simulink model "WHEELSPEEDTEST"  (R2024b)
settings: Solver=ode4  StartTime=0.0  StopTime=T_SIM  FixedStep=T_s  RelTol=1e-3
values from neighbouring files (symbols this model uses):
  control_par = [1.5, 1.5, 0.3]    [TASK1_Script.m]    (also in TASK2_LAB_SCRIPT.m = update_control_par(controller_index); TASK2_Scirpt.m = [k1, k2,b]; TASK3_Script.m = [k1, k2,b])
  d = d_actual    (= 0.1604)    [TASK1_Script.m]    (also in TASK2_LAB_SCRIPT.m; TASK2_Scirpt.m; TASK3_Script.m)
  D = diag([0.8e-3, 0.8e-3, 5e-3, 0.0175/6, 0.0175/6, 0.0175/6*T_s, 0.0175/6*T_s].^2)    [TASK1_Script.m]    (also in TASK2_LAB_SCRIPT.m; TASK2_Scirpt.m; TASK3_Script.m)
  d_actual = 0.16040    (= 0.1604)    [TASK1_Script.m]    (also in TASK2_LAB_SCRIPT.m; TASK2_Scirpt.m; TASK3_Script.m)
  H_enc = [0, 0, 0, 1, 0, 0, 0 ... (first row only)    [TASK1_Script.m]    (also in TASK2_LAB_SCRIPT.m; TASK2_Scirpt.m; TASK3_Script.m)
  H_gyro = [0, 0, 0, 0, 0, -r_actual/d_actual, r_actual/d_actual]    [TASK1_Script.m]    (also in TASK2_LAB_SCRIPT.m; TASK2_Scirpt.m; TASK3_Script.m)
  H_motion_cap = [1, 0, 0, 0, 0, 0, 0 ... (first row only)    [TASK1_Script.m]    (also in TASK2_LAB_SCRIPT.m; TASK2_Scirpt.m; TASK3_Script.m)
  omega_M = 10    [TASK1_Script.m]    (also in TASK2_LAB_SCRIPT.m; TASK2_Scirpt.m; TASK3_Script.m)
  P_INIT_EKF = diag([0.1, 0.1, 0.2, 0.0175/6, 0.0175/6, 0.0175/6*T_s, 0.0175/6*T_s].^2)    [TASK1_Script.m]    (also in TASK2_LAB_SCRIPT.m; TASK2_Scirpt.m; TASK3_Script.m)
  p_loss = 0.9    [TASK3_Script.m]
  PHI_INIT = [0;0]    [TASK1_Script.m]    (also in TASK2_LAB_SCRIPT.m; TASK2_Scirpt.m; TASK3_Script.m)
  q_d = [-1.6; -1.1; 0]    [TASK1_Script.m]
  Q_INIT = Q_INIT_1    [TASK1_Script.m]    (also in TASK2_LAB_SCRIPT.m = [-1.6;-1.1;0]; TASK2_Scirpt.m = [-1.6;-1.1;0]; TASK3_Script.m = [x7; y4; 0])
  r = r_actual    (= 0.03293)    [TASK1_Script.m]    (also in TASK2_LAB_SCRIPT.m; TASK2_Scirpt.m; TASK3_Script.m)
  R_3 = diag(([sigma_motion_capture, sigma_motion_capture, sigma_motion_capture,               sigma_enc, sigma_enc, sigma_imu]).^2)    [TASK1_Script.m]    (also in TASK2_LAB_SCRIPT.m; TASK2_Scirpt.m; TASK3_Script.m)
  r_actual = 0.03293    [TASK1_Script.m]    (also in TASK2_LAB_SCRIPT.m; TASK2_Scirpt.m; TASK3_Script.m)
  T_s = 0.04    [TASK1_Script.m]    (also in TASK2_LAB_SCRIPT.m; TASK2_Scirpt.m; TASK3_Script.m; plot_4_wheel_velocities.m)
  tol = 0.025    [TASK1_Script.m]
  Z_INIT_EKF = [Q_INIT; 0; 0; 0; 0]    [TASK1_Script.m]    (also in TASK2_LAB_SCRIPT.m; TASK2_Scirpt.m; TASK3_Script.m)
undefined symbols (not defined in the file or in its folder): X, Y
libraries: robotlib x6, sharedtransform x2, dspsigops x1
settings Model: Creator=tomailoren  LastModifiedBy=llp
settings OptimizationCC: DefaultParameterBehavior=Inlined  EnhancedBackFolding=on  PassReuseOutputArgsAs=Individual arguments  ZeroExternalMemoryAtStartup=off  ZeroInternalMemoryAtStartup=off  MaxStackSize=64  OptimizeBlockOrder=speed  DifferentSizesBufferReuse=on  OptimizationCustomize=off  EfficientTunableParamExpr=on
settings DebuggingCC: ParameterTunabilityLossMsg=error
settings HardwareCC: ProdBitPerPointer=32  ProdBitPerSizeT=32  ProdBitPerPtrDiffT=32  ProdLargestAtomicFloat=None  ProdIntDivRoundTo=Undefined  ProdEndianess=Unspecified  ProdWordSize=32  ProdHWDeviceType=Generic->Unspecified (assume 32-bit Generic)
settings SFSimCC: MATLABDynamicMemAlloc=off
settings RTWCC: Description=Embedded Coder  SystemTargetFile=ert.tlc  HardwareBoard=Robot Operating System (ROS)  TLCOptions="-aInlineSetEventsForThisBaseRateFcn=TLC_FALSE -aSuppressMultiTaskScheduler=TLC_FALSE  -aRateBasedStepFcn=0"  TemplateMakefile=ert_default_tmf  Toolchain=Catkin  TargetLang=C++
settings CodeAppCC: ForceParamTrailComments=on  IgnoreCustomStorageClasses=off  OperatorAnnotations=on  SimulinkDataObjDesc=on  SFDataObjDesc=on  InsertBlockDesc=on

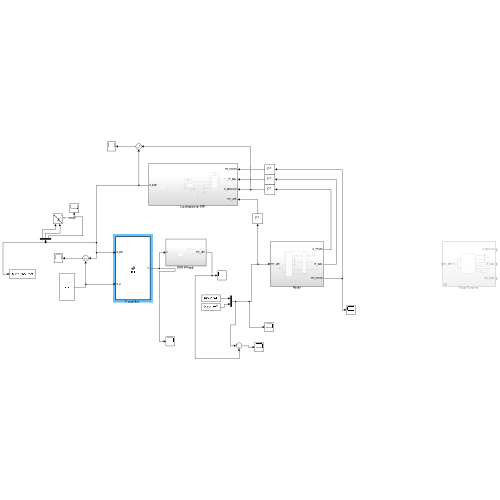
[thumbnail: Simulink's stored preview of the top-level diagram]
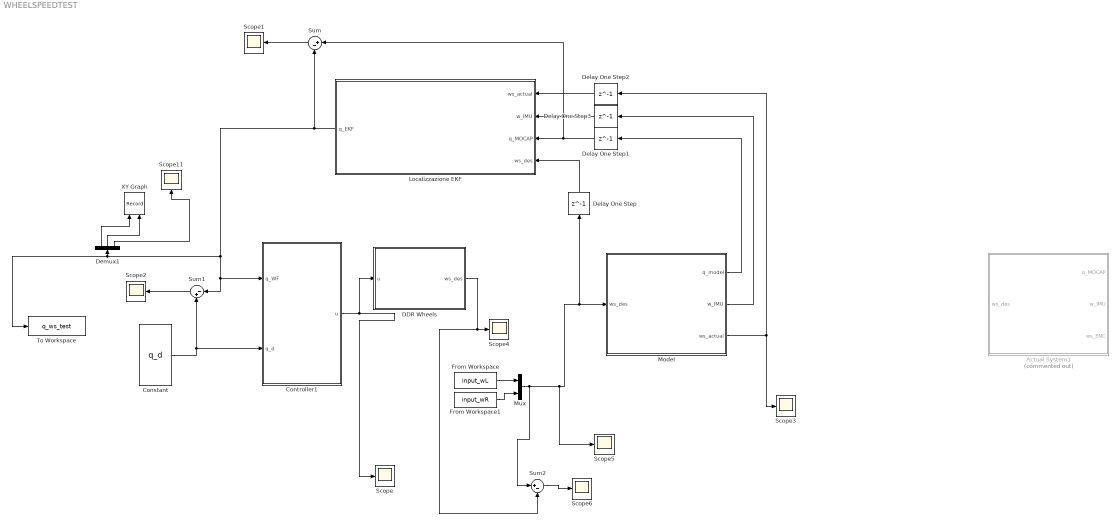
== system WHEELSPEEDTEST ==
  Actual System1 : Subsystem  Commented=on
  Constant : Constant  Value=q_d
  Controller1 : MATLAB Function  TreatAsAtomicUnit=on
  DDR Wheels : Subsystem
  Delay One Step : Delay  DelayLength=1  InitialCondition=[0;0]  SampleTime=T_s
  Delay One Step1 : Delay  DelayLength=1  InitialCondition=Q_INIT  SampleTime=T_s
  Delay One Step2 : Delay  DelayLength=1  InitialCondition=[0;0]  SampleTime=T_s
  Delay One Step3 : Delay  DelayLength=1  InitialCondition=0  SampleTime=T_s
  Demux1 : Demux  Outputs=3
  From Workspace : FromWorkspace  VariableName=input_wL
  From Workspace1 : FromWorkspace  VariableName=input_wR
  Localizzazione EKF : Subsystem
  Model : Subsystem
  Mux : Mux  Inputs=2
  Scope{,1..6,11} (8 alike) : Scope
  Sum : Sum  Inputs=|+-
  Sum1 : Sum  Inputs=|-+
  Sum2 : Sum  Inputs=|+-
  To Workspace : ToWorkspace  VariableName=q_ws_test  SaveFormat=Structure With Time  SampleTime=-1
  XY Graph : Record  FileSettingsInternal="{\"entries\":[{\"content\":{\"excelSettings\":{\"content\":{},\"type\":\"Streamout.ExcelSettings\"}},\"type\":\"Streamout.FileSettingStorage\",\"uuid\":\"\"}],\"packageUris\":[\"http:\\/\\/schema.mathworks.com\\/mf0\\/streamout_blocks\\/R2020a\"],\"version\":\"1.0\"}"  Layout=[1 1]  SignalsInternal="{\"entries\":[{\"content\":{\"signals\":[{\"content\":{\"blockPath\":[],\"dimensions\":[1,1],\"domain\":\"\",\"lineColor\":\"#a2142f\",\"plots\":[ 1 ],\"port\":1,\"signalID\":1,\"signalName\":\"Demux1:1\"},\"type\":\"RecordBlkView.Signal\",\"uuid\":\"\"},{\"content\":{\"blockPath\":[],\"dimensions\":[1,1],\"domain\":\"\",\"lineColor\":\"#139fff\",\"plots\":[ 1 ],\"port\":2,\"signalID\":2,\"signalName\":\"Demux1:2\"},\"type\":\"RecordBlkView.Signal\",\"uuid\":\"\"}]},\"type\":\"RecordBlkView.InputSignals\",\"uuid\":\"\"}],\"packageUris\":[\"http:\\/\\/schema.mathworks.com\\/mf0\\/streamout_blocks\\/R2020a\"],\"version\":\"1.0\"}"  VisualizationBindings="{\"xyplotplugin\":{\"info\":[{\"series\":[{\"bindingParametersList\":[{\"parameter\":\"X-Axis\",\"signalID\":1,\"signalName\":\"Demux1:1\"},{\"parameter\":\"Y-Axis\",\"signalID\":2,\"signalName\":\"Demux1:2\"}],\"seriesID\":0}],\"subplotID\":1}]}}"  CompatibilityTag=XY
  wires:
  Controller1/1(u) -> Scope/1, DDR Wheels/1(u)
  Localizzazione EKF/1(q_EKF) -> Sum/2, Sum1/1, Controller1/1(q_WF), To Workspace/1, Demux1/1
  Model/1(q_model) -> Delay One Step1/1
  Model/3(ws_actual) -> Scope3/1, Delay One Step2/1
  Model/2(w_IMU) -> Delay One Step3/1
  Delay One Step/1 -> Localizzazione EKF/4(ws_des)
  Constant/1 -> Sum1/2, Controller1/2(q_d)
  Demux1/1 -> XY Graph/1
  Demux1/2 -> XY Graph/2
  Demux1/3 -> Scope11/1
  Delay One Step1/1 -> Sum/1, Localizzazione EKF/3(q_MOCAP)
  Delay One Step2/1 -> Localizzazione EKF/1(ws_actual)
  Delay One Step3/1 -> Localizzazione EKF/2(w_IMU)
  Sum/1 -> Scope1/1
  Sum1/1 -> Scope2/1
  DDR Wheels/1(ws_des) -> Sum2/2, Scope4/1
  Mux/1 -> Sum2/1, Scope5/1, Delay One Step/1, Model/1(ws_des)
  From Workspace/1 -> Mux/1
  From Workspace1/1 -> Mux/2
  Sum2/1 -> Scope6/1

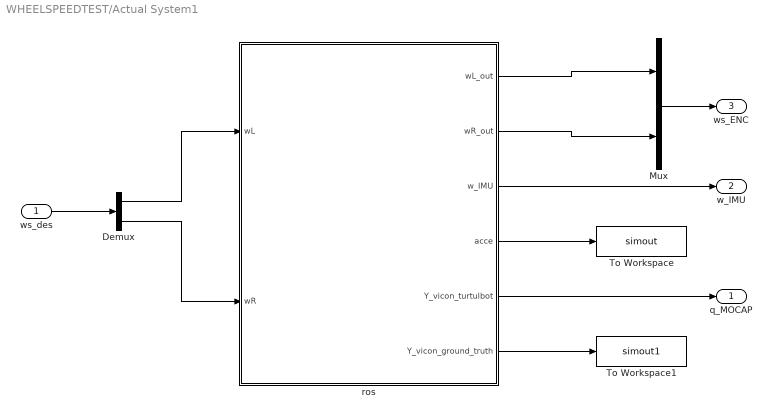
== system WHEELSPEEDTEST/Actual System1 ==
  ws_des : Inport
  Demux : Demux  Outputs=2
  Mux : Mux  Inputs=2
  To Workspace : ToWorkspace  VariableName=simout  SaveFormat=Timeseries  SampleTime=-1
  To Workspace1 : ToWorkspace  VariableName=simout1  SaveFormat=Timeseries  SampleTime=-1
  ros : Subsystem
  q_MOCAP : Outport
  w_IMU : Outport  Port=2
  ws_ENC : Outport  Port=3
  wires:
  ros/2(wR_out) -> Mux/2
  ros/4(acce) -> To Workspace/1
  ros/5(Y_vicon_turtulbot) -> q_MOCAP/1
  ros/1(wL_out) -> Mux/1
  ros/3(w_IMU) -> w_IMU/1
  ws_des/1 -> Demux/1
  Demux/1 -> ros/1(wL)
  Demux/2 -> ros/2(wR)
  Mux/1 -> ws_ENC/1
  ros/6(Y_vicon_ground_truth) -> To Workspace1/1

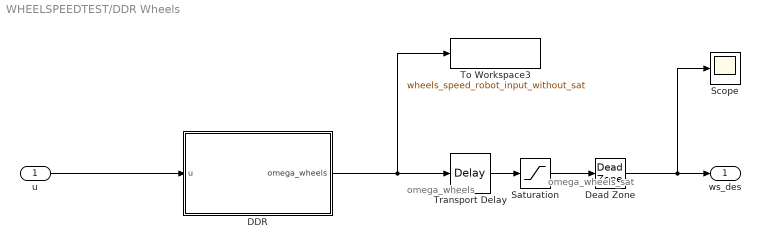
== system WHEELSPEEDTEST/DDR Wheels ==
  note: omega_wheels_sat
  note: omega_wheels
  u : Inport
  DDR : MATLAB Function  TreatAsAtomicUnit=on
  Dead Zone : DeadZone  LowerValue=-0.1  UpperValue=0.1
  Saturation : Saturate  UpperLimit=omega_M  LowerLimit=-omega_M
  Scope : Scope
  To Workspace3 : ToWorkspace  VariableName=wheels_speed_robot_input_without_sat  SaveFormat=Structure With Time  SampleTime=-1
  Transport Delay : TransportDelay  DelayTime=0.09
  ws_des : Outport
  wires:
  DDR/1(omega_wheels) -> To Workspace3/1, Transport Delay/1
  Saturation/1 -> Dead Zone/1
  u/1 -> DDR/1(u)
  Transport Delay/1 -> Saturation/1
  Dead Zone/1 -> Scope/1, ws_des/1

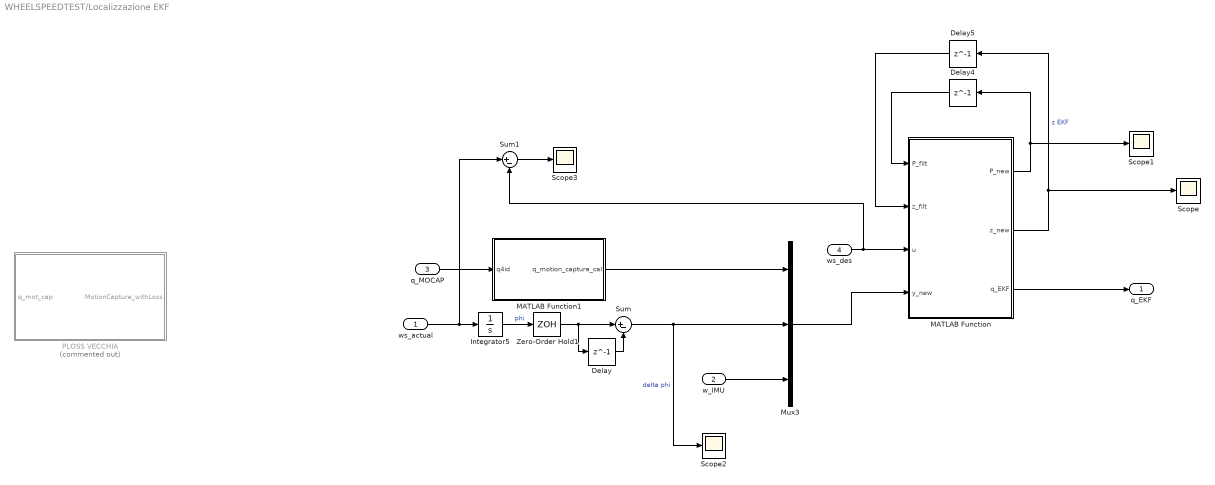
== system WHEELSPEEDTEST/Localizzazione EKF ==
  ws_actual : Inport
  w_IMU : Inport  Port=2
  q_MOCAP : Inport  Port=3
  ws_des : Inport  Port=4
  Delay : Delay  DelayLength=1  InitialCondition=[0;0]  SampleTime=T_s
  Delay4 : Delay  DelayLength=1  InitialCondition=P_INIT_EKF  SampleTime=T_s
  Delay5 : Delay  DelayLength=1  InitialCondition=Z_INIT_EKF  SampleTime=T_s
  Integrator5 : Integrator  InitialCondition=PHI_INIT
  MATLAB Function : MATLAB Function  TreatAsAtomicUnit=on
  MATLAB Function1 : MATLAB Function  TreatAsAtomicUnit=on
  Mux3 : Mux  Inputs=3
  PLOSS VECCHIA : Subsystem  Commented=on
  Scope{,1..3} (4 alike) : Scope
  Sum : Sum  Inputs=|+-
  Sum1 : Sum  Inputs=|+-
  Zero-Order Hold1 : ZeroOrderHold  SampleTime=T_s
  q_EKF : Outport
  wires:
  MATLAB Function/2(z_new) -> Scope/1, Delay5/1  "z EKF"
  Delay5/1 -> MATLAB Function/2(z_filt)
  q_MOCAP/1 -> MATLAB Function1/1(q4id)
  w_IMU/1 -> Mux3/3
  Delay4/1 -> MATLAB Function/1(P_filt)
  MATLAB Function/1(P_new) -> Scope1/1, Delay4/1
  ws_des/1 -> MATLAB Function/3(u), Sum1/2
  MATLAB Function1/1(q_motion_capture_cal) -> Mux3/1
  Mux3/1 -> MATLAB Function/4(y_new)
  MATLAB Function/3(q_EKF) -> q_EKF/1
  Sum/1 -> Scope2/1, Mux3/2  "delta phi"
  Zero-Order Hold1/1 -> Delay/1, Sum/1
  ws_actual/1 -> Sum1/1, Integrator5/1
  Integrator5/1 -> Zero-Order Hold1/1  "phi"
  Delay/1 -> Sum/2
  Sum1/1 -> Scope3/1

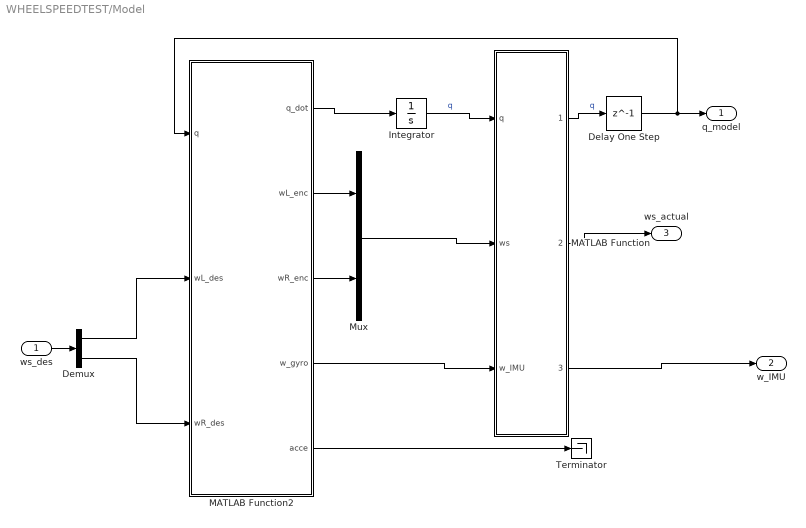
== system WHEELSPEEDTEST/Model ==
  ws_des : Inport
  Delay One Step : Delay  DelayLength=1  InitialCondition=Q_INIT
  Demux : Demux  Outputs=2
  Integrator : Integrator  InitialCondition=Q_INIT
  MATLAB Function : MATLAB Function  TreatAsAtomicUnit=on
  MATLAB Function2 : MATLAB Function  TreatAsAtomicUnit=on
  Mux : Mux  Inputs=2
  Terminator : Terminator
  q_model : Outport
  w_IMU : Outport  Port=2
  ws_actual : Outport  Port=3
  wires:
  MATLAB Function/1(q_noise) -> Delay One Step/1  "q"
  Demux/1 -> MATLAB Function2/2(wL_des)
  Demux/2 -> MATLAB Function2/3(wR_des)
  MATLAB Function2/5(acce) -> Terminator/1
  ws_des/1 -> Demux/1
  MATLAB Function2/2(wL_enc) -> Mux/1
  MATLAB Function2/3(wR_enc) -> Mux/2
  Mux/1 -> MATLAB Function/2(ws)
  MATLAB Function2/4(w_gyro) -> MATLAB Function/3(w_IMU)
  MATLAB Function/2(ws_noise) -> ws_actual/1
  MATLAB Function/3(w_IMU_noise) -> w_IMU/1
  MATLAB Function2/1(q_dot) -> Integrator/1
  Integrator/1 -> MATLAB Function/1(q)  "q"
  Delay One Step/1 -> MATLAB Function2/1(q), q_model/1

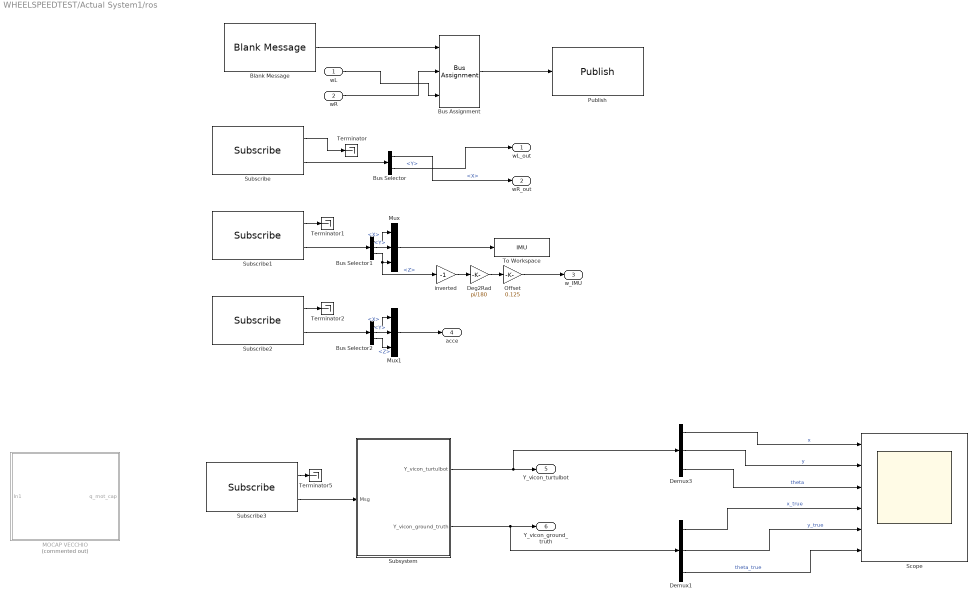
== system WHEELSPEEDTEST/Actual System1/ros ==
  wL : Inport
  wR : Inport  Port=2
  Blank Message : robotlib/Blank Message  messageClass=Message  entityType=geometry_msgs/Vector3  messageType=geometry_msgs/Vector3  SampleTime=T_s  legacyBusStruct=off
  Bus Assignment : BusAssignment  AssignedSignals=X,Y
  Bus Selector : BusSelector  OutputSignals=X,Y
  Bus Selector1 : BusSelector  OutputSignals=X,Y,Z
  Bus Selector2 : BusSelector  OutputSignals=X,Y,Z
  Deg2Rad : Gain  Gain=pi/180
  Demux1 : Demux  Outputs=3
  Demux3 : Demux  Outputs=3
  MOCAP VECCHIO : Subsystem  Commented=on
  Mux : Mux  Inputs=3
  Mux1 : Mux  Inputs=3
  Offset : Gain  Gain=0.125
  Publish : robotlib/Publish  topicSource=Select from ROS network  topic=/turtlebot_01/cmd_wheels  messageType=geometry_msgs/Vector3  legacyBusStruct=off  messageQueueLength=1
  Scope : Scope  NumInputPorts=6
  Subscribe : robotlib/Subscribe  topicSource=Select from ROS network  topic=/turtlebot_01/wheelSpeeds  messageType=geometry_msgs/Vector3  SampleTime=T_s  legacyBusStruct=off  messageQueueLength=1
  Subscribe1 : robotlib/Subscribe  topicSource=Select from ROS network  topic=/turtlebot_01/gyroscope  messageType=geometry_msgs/Vector3  SampleTime=T_s  legacyBusStruct=off  messageQueueLength=1
  Subscribe2 : robotlib/Subscribe  topicSource=Select from ROS network  topic=/turtlebot_01/accelerometer  messageType=geometry_msgs/Vector3  SampleTime=T_s  legacyBusStruct=off  messageQueueLength=1
  Subscribe3 : robotlib/Subscribe  topicSource=Select from ROS network  topic=/turtlebot_01/odom  messageType=nav_msgs/Odometry  SampleTime=T_s  legacyBusStruct=off  messageQueueLength=1
  Subsystem : Subsystem
  Terminator{,1..2,5} (4 alike) : Terminator
  To Workspace : ToWorkspace  VariableName=IMU  SaveFormat=Structure With Time  SampleTime=-1
  inverted : Gain  Gain=-1
  wL_out : Outport
  wR_out : Outport  Port=2
  w_IMU : Outport  Port=3
  acce : Outport  Port=4
  Y_vicon_turtulbot : Outport  Port=5
  Y_vicon_ground_truth : Outport  Port=6
  wires:
  Subscribe2/2 -> Bus Selector2/1
  wR/1 -> Bus Assignment/2
  Bus Selector/1 -> wR_out/1  "<X>"
  Bus Selector1/2 -> Mux/2  "<Y>"
  Bus Selector2/2 -> Mux1/2  "<Y>"
  Bus Selector2/1 -> Mux1/1  "<X>"
  Bus Assignment/1 -> Publish/1
  Subscribe2/1 -> Terminator2/1
  inverted/1 -> Deg2Rad/1
  Subscribe3/1 -> Terminator5/1
  Subscribe/2 -> Bus Selector/1
  Mux1/1 -> acce/1
  Deg2Rad/1 -> Offset/1
  Bus Selector1/3 -> inverted/1, Mux/3  "<Z>"
  Offset/1 -> w_IMU/1
  wL/1 -> Bus Assignment/3
  Bus Selector1/1 -> Mux/1  "<X>"
  Bus Selector2/3 -> Mux1/3  "<Z>"
  Mux/1 -> To Workspace/1
  Subscribe/1 -> Terminator/1
  Bus Selector/2 -> wL_out/1  "<Y>"
  Subscribe1/2 -> Bus Selector1/1
  Subscribe1/1 -> Terminator1/1
  Blank Message/1 -> Bus Assignment/1
  Subscribe3/2 -> Subsystem/1(Msg)
  Demux1/2 -> Scope/5  "y_true"
  Subsystem/1(Y_vicon_turtulbot) -> Demux3/1, Y_vicon_turtulbot/1
  Subsystem/2(Y_vicon_ground_truth) -> Y_vicon_ground_truth/1, Demux1/1
  Demux3/3 -> Scope/3  "theta"
  Demux1/1 -> Scope/4  "x_true"
  Demux3/1 -> Scope/1  "x"
  Demux1/3 -> Scope/6  "theta_true"
  Demux3/2 -> Scope/2  "y"

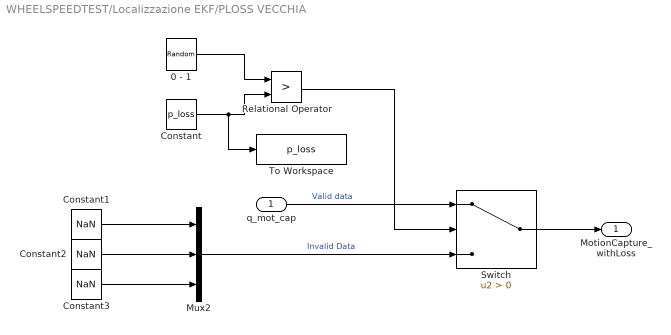
== system WHEELSPEEDTEST/Localizzazione EKF/PLOSS VECCHIA ==
  q_mot_cap : Inport
  0 - 1 : UniformRandomNumber  Minimum=0  SampleTime=T_s
  Constant : Constant  Value=p_loss
  Constant1 : Constant  Value=NaN
  Constant2 : Constant  Value=NaN
  Constant3 : Constant  Value=NaN
  Mux2 : Mux  Inputs=3
  Relational Operator : RelationalOperator  Operator=>  OutDataTypeStr=boolean  RndMeth=Simplest  InputSameDT=off
  Switch : Switch  Criteria=u2 > Threshold  SaturateOnIntegerOverflow=off  InputSameDT=off
  To Workspace : ToWorkspace  VariableName=p_loss  SaveFormat=Structure  SampleTime=-1
      settings: Save2DSignal=2-D array (concatenate along first dimension)
  MotionCapture_withLoss : Outport
  wires:
  0 - 1/1 -> Relational Operator/1
  Constant/1 -> To Workspace/1, Relational Operator/2
  Switch/1 -> MotionCapture_withLoss/1
  Relational Operator/1 -> Switch/2
  Constant2/1 -> Mux2/2
  Mux2/1 -> Switch/3  "Invalid Data"
  Constant1/1 -> Mux2/1
  q_mot_cap/1 -> Switch/1  "Valid data"
  Constant3/1 -> Mux2/3

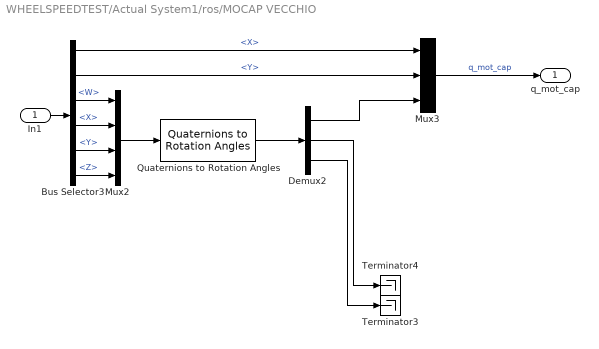
== system WHEELSPEEDTEST/Actual System1/ros/MOCAP VECCHIO ==
  In1 : Inport
  Bus Selector3 : BusSelector  OutputSignals=Pose.Pose.Position.X,Pose.Pose.Position.Y,Pose.Pose.Orientation.W,Pose.Pose.Orientation.X,Pose.Pose.Orientation.Y,Pose.Pose.Orientation.Z
  Demux2 : Demux  Outputs=3
  Mux2 : Mux
  Mux3 : Mux  Inputs=3
  Quaternions to Rotation Angles : sharedtransform/Quaternions to Rotation Angles  rotationOrder=ZYX  aMode=aMode
  Terminator3 : Terminator
  Terminator4 : Terminator
  q_mot_cap : Outport
  wires:
  Bus Selector3/3 -> Mux2/1  "<W>"
  Demux2/2 -> Terminator4/1
  Quaternions to Rotation Angles/1 -> Demux2/1
  Mux3/1 -> q_mot_cap/1  "q_mot_cap"
  Bus Selector3/4 -> Mux2/2  "<X>"
  Demux2/1 -> Mux3/3
  Mux2/1 -> Quaternions to Rotation Angles/1
  Bus Selector3/1 -> Mux3/1  "<X>"
  Demux2/3 -> Terminator3/1
  Bus Selector3/2 -> Mux3/2  "<Y>"
  Bus Selector3/5 -> Mux2/3  "<Y>"
  Bus Selector3/6 -> Mux2/4  "<Z>"
  In1/1 -> Bus Selector3/1

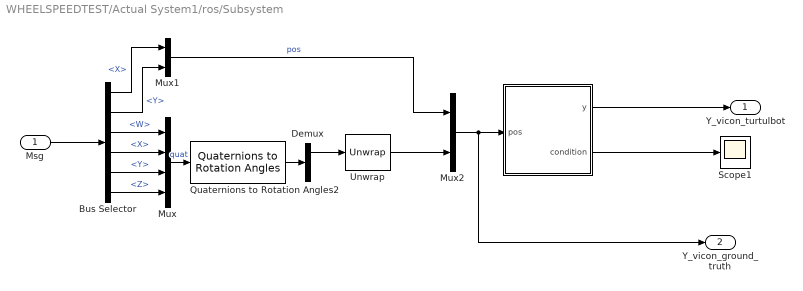
== system WHEELSPEEDTEST/Actual System1/ros/Subsystem ==
  Msg : Inport
  " " : MATLAB Function  TreatAsAtomicUnit=on
  Bus Selector : BusSelector  OutputSignals=Pose.Pose.Position.X,Pose.Pose.Position.Y,Pose.Pose.Orientation.W,Pose.Pose.Orientation.X,Pose.Pose.Orientation.Y,Pose.Pose.Orientation.Z
  Demux : Demux  Outputs=3
  Mux : Mux
  Mux1 : Mux  Inputs=2
  Mux2 : Mux  Inputs=2
  Quaternions to Rotation Angles2 : sharedtransform/Quaternions to Rotation Angles  rotationOrder=ZYX  aMode=aMode
  Scope1 : Scope
  Unwrap : dspsigops/Unwrap  tol=pi  InputProcessing=Columns as channels (frame based)  running=off
  Y_vicon_turtulbot : Outport
  Y_vicon_ground_truth : Outport  Port=2
  wires:
  Msg/1 -> Bus Selector/1
  Mux2/1 -> Y_vicon_ground_truth/1, " "/1(pos)
  Bus Selector/3 -> Mux/1  "<W>"
  Mux/1 -> Quaternions to Rotation Angles2/1  "quat"
  Bus Selector/2 -> Mux1/2  "<Y>"
  Bus Selector/6 -> Mux/4  "<Z>"
  Bus Selector/1 -> Mux1/1  "<X>"
  " "/1(y) -> Y_vicon_turtulbot/1
  Bus Selector/4 -> Mux/2  "<X>"
  Bus Selector/5 -> Mux/3  "<Y>"
  " "/2(condition) -> Scope1/1
  Unwrap/1 -> Mux2/2
  Mux1/1 -> Mux2/1  "pos"
  Quaternions to Rotation Angles2/1 -> Demux/1
  Demux/1 -> Unwrap/1

== matlab function WHEELSPEEDTEST/DDR Wheels/DDR ==
  data: u input; omega_wheels output; r parameter; d parameter
function omega_wheels = kin2omegawheels(u, r, d)
omega_l = u(1)/r-d/(2*r)*u(2);
omega_r = u(1)/r+d/(2*r)*u(2);
omega_wheels = [omega_l;omega_r];

== matlab function WHEELSPEEDTEST/Model/MATLAB Function ==
  settings: updateMethod=DISCRETE
  data: q input; q_noise output; ws input; w_IMU input; ws_noise output; w_IMU_noise output; D parameter
function [q_noise, ws_noise, w_IMU_noise] = fcn(q, ws, w_IMU, D)

    % --- DEVIAZIONI STANDARD (sigma) ---
    
    % Deviazioni per il modello (q)
    sigma_x     = D(1,1); 
    sigma_y     = D(2,2);
    sigma_theta = D(3,3); 
    sigma_ws    = D(6,6); 
    sigma_w_IMU = 0.01;      
    % sigma_x     = 5e-3; 
    % sigma_y     = 5e-3;
    % sigma_theta = 5e-2; 
    % sigma_ws    = 1e-1; 
    % sigma_w_IMU = 2e-2;
    
    % --- GENERAZIONE RUMORE STATO (q) ---
    % Moltiplica per sigma, non per sigma^2
    x_n = q(1) + sigma_x * randn;
    y_n = q(2) + sigma_y * randn;
    
    % Prima aggiungi il rumore, POI wrappi l'angolo
    theta_noisy = q(3) + sigma_theta * randn;
    theta_n = atan2(sin(theta_noisy), cos(theta_noisy));
    
    q_noise = [x_n; y_n; theta_n];
    
    % --- GENERAZIONE RUMORE SENSORI ---
    ws_noise    = ws    + sigma_ws    * randn(size(ws));
    w_IMU_noise = w_IMU + sigma_w_IMU * randn(size(w_IMU));

end

== matlab function WHEELSPEEDTEST/Localizzazione EKF/MATLAB Function1 ==
  data: q4id input; q_motion_capture_cal output
function q_motion_capture_cal = calibration(q4id)

x_off_cal = -0.00434;
y_off_cal = -0.00361;
theta_off = 0.02331;


theta_cal = q4id(3) - theta_off;
x_cal = q4id(1) - (x_off_cal * cos(theta_cal) - y_off_cal * sin(theta_cal));
y_cal = q4id(2) - (x_off_cal * sin(theta_cal) + y_off_cal * cos(theta_cal));


q_motion_capture_cal = [x_cal; y_cal; theta_cal];

== matlab function WHEELSPEEDTEST/Model/MATLAB Function2 ==
  data: q input; q_dot output; wL_des input; wR_des input; wL_enc output; wR_enc output; w_gyro output; r parameter; d parameter; T_s parameter; acce output
function [q_dot, wL_enc, wR_enc, w_gyro, acce] = robot_simulator(q, wL_des, wR_des, r, d, T_s)
    
    wL_enc = wL_des;
    wR_enc = wR_des;
      
    v = (r/2) * (wR_des + wL_des);
    omega = (r/d) * (wR_des - wL_des);
    
    w_gyro = -omega;
    
    q_dot= zeros(3,1);
    
    q_dot(1) = v*cos(q(3));
    q_dot(2) = v*sin(q(3));
    q_dot(3) = omega;

    acce = [0;0;0];
    
end

== matlab function WHEELSPEEDTEST/Actual System1/ros/Subsystem/  ==
  data: y output; pos input; condition output
function [y, condition] = check(pos)

x1 = -2.9; y1 = -1.5;
x2 = -1.6; y2 = -1.1;
x3 = -1.5; y3 = -0.7;
x4 = -1.4; y4 = -0.3;
x5 = -0.6; y5 =  0.1;
x6 =  0.2; y6 =  1.5;
x7 =  1.0;
x8 =  1.1;
x9 =  2.9;

P_loss = 0.9;


if ((pos(1) >= x5) && (pos(1) <= x6)) && ((pos(2) >= y1) && (pos(2) <= y5))
    % add noise
    y = pos + 0.02*randn(3,1);
    condition = 1;
elseif ((pos(1) >= x7) && (pos(1) <= x9)) && ((pos(2) >= y1) && (pos(2) <= y6))
    % measurement loss
    if rand > P_loss
        y = pos;
    else
        y = 0*pos;
    end
    condition = 2;
else
    y = pos;
    condition = 0;
end

== matlab function WHEELSPEEDTEST/Localizzazione EKF/MATLAB Function ==
  data: P_filt input; P_new output; z_filt input; z_new output; u input; y_new input; D parameter; T_s parameter; r_actual parameter; d_actual parameter; H_enc parameter; H_gyro parameter; H_motion_cap parameter; R_3 parameter; q_EKF output
function [P_new, z_new, q_EKF] = EKF_filtering(P_filt, z_filt, u, y_new, D, T_s, r_actual, d_actual, H_enc, H_gyro, H_motion_cap, R_3)

    % Def state z_filt: [xk , yk , thetak , delta_phi_L_km1 , delta_phi_R_km1 , wLk , wRk ]

    r = r_actual;
    d = d_actual;
        
    % Extraction variables
    x_k = z_filt(1);
    y_k = z_filt(2);
    theta_k = z_filt(3);
    delta_phi_L_km1 = z_filt(4);
    delta_phi_R_km1 = z_filt(5); 
    wL_k = z_filt(6);               % estimate wheels velocities
    wR_k = z_filt(7);
    
    uL_k = u(1);                    % actual wheels velocities (from command input v,w)
    uR_k = u(2);

    % ----------------------

    % PREDICT STEP
    v_k = (r/2) * (wL_k + wR_k);
    omega_k = (r/d) * (wR_k - wL_k);
    theta_mean = theta_k + (omega_k * T_s) / 2;
        
    % State Prediction (approximation with RK2)
    x_kp1 = x_k + v_k * T_s * cos(theta_mean);
    y_kp1 = y_k + v_k * T_s * sin(theta_mean);
    theta_kp1 = theta_k + omega_k * T_s;

    theta_kp1 = atan2(sin(theta_kp1), cos(theta_kp1));
    
    delta_phi_L_k = wL_k * T_s;
    delta_phi_R_k = wR_k * T_s;
    
    wL_kp1 = uL_k; 
    wR_kp1 = uR_k;
    
    z_hat = [x_kp1; y_kp1; theta_kp1; delta_phi_L_k; delta_phi_R_k; wL_kp1; wR_kp1];
    
    % F derivation
    F = zeros(7,7);
    
    F(1,1) = 1;
    F(1, 3) = -T_s * v_k * sin(theta_mean);
    F(1, 6) = (T_s * r / 2) * cos(theta_mean) - v_k * T_s * sin(theta_mean) * (-T_s * r / (2 * d));
    F(1, 7) = (T_s * r / 2) * cos(theta_mean) - v_k * T_s * sin(theta_mean) * (T_s * r / (2 * d));
    
    F(2,2) = 1;
    F(2, 3) = v_k * T_s * cos(theta_mean);
    F(2, 6) = (T_s * r / 2) * sin(theta_mean) + v_k * T_s * cos(theta_mean) * (-T_s * r / (2 * d));
    F(2, 7) = (T_s * r / 2) * sin(theta_mean) + v_k * T_s * cos(theta_mean) * (T_s * r / (2 * d));

    F(3,3) = 1;
    F(3, 6) = -T_s * r / d;
    F(3, 7) = T_s * r / d;

    F(4, 6) = T_s;
    F(5, 7) = T_s;
    
    % Covariance Prediction
    P_hat = F * P_filt * F' + D;
    
    % ----------------------

    % UPDATE STEP
    % H and R will depend on the measurement data y_new and Test_case

    % enc_values (delta_phi)
    % IMU_values (w_gyro)
    % Motion_capture (state q)

    % y_new = [x; y; theta; delta_phi_L; delta_phi_R; omega_gyro]

    %% OBSERVATION MATRIX H ALWAYS FULL (6X7) AND ALSO Y_NEW (6X1) 
    H_full = [H_motion_cap; H_enc; H_gyro];
    y_meas = y_new; 
    
    % Start with full matrix R_3 
    R_current = R_3;
    INFINITY_VAR = 1e9; % Infinite var to put down the Kalman gain

    % IMU not available
    R_current(6,6) = INFINITY_VAR;
    
    % TEST 3: all active, possibile data loss
    if any(isnan(y_new(1:3)))   
        y_meas(1:3) = 0;    % force to zero just for completness
        R_current(1,1) = INFINITY_VAR; 
        R_current(2,2) = INFINITY_VAR; 
        R_current(3,3) = INFINITY_VAR;
    end

    
    % Innovation e_pred
    y_hat = H_full * z_hat;
    e_kp1 = y_meas - y_hat;

    e_kp1(3) = atan2(sin(e_kp1(3)), cos(e_kp1(3)));
    
    % Kalman Gain K_pred
    K = P_hat * H_full' / (H_full * P_hat * H_full' + R_current);   
    
    % State and Covariance Update
    z_new = z_hat + K * e_kp1;

    z_new(3) = atan2(sin(z_new(3)), cos(z_new(3)));
    
    P_new = P_hat - K * H_full * P_hat;


    q_EKF = z_new(1:3);

end

== matlab function WHEELSPEEDTEST/Controller1 ==
  data: q_WF input; q_d input; u output; control_par parameter; tol parameter
function u = fcn(q_WF, q_d, control_par,tol)
% select the controller
k1 = control_par(1);
k2 = control_par(2);
k3 = control_par(3);

xd = q_d(1);
yd = q_d(2);
thetad = q_d(3);


e = q_WF-q_d;

x_t = cos(thetad)*e(1)+sin(thetad)*e(2);
y_t = -sin(thetad)*e(1)+cos(thetad)*e(2);
theta_t = e(3);

rho = sqrt(x_t^2+y_t^2);
%gamma = atan2(y_t,x_t)+pi-theta_t;
%delta = theta_t +gamma;

%v = k1*rho*cos(gamma);
%omega = k2*gamma + k1 *(sin(gamma)*cos(gamma))/gamma *(gamma+k3*delta);

%u = [v;omega];

    if rho < tol
        v = 0;
        omega = 0;
    else
        % --- CALCOLO DEL CONTROLLO NORMALE ---
        gamma = atan2(y_t, x_t) + pi - theta_t;
        delta = theta_t + gamma;
        
        v = k1 * rho * cos(gamma);
        
        % Protezione contro la divisione per zero quando gamma è piccolissimo
        if abs(gamma) < 1e-1
            term_gamma = 1; 
        else
            term_gamma = (sin(gamma)*cos(gamma))/gamma;
        end
        
        omega = k2*gamma + k1 * term_gamma * (gamma + k3*delta);
    end
    
    u = [v; omega];

end
